simulink model "filter0"  (R2020b)
settings: Solver=FixedStepAuto  StartTime=0.0  StopTime=10.0  FixedStep=0.5  RelTol=1e-3
settings Model: Creator=Puru Gawande  LastModifiedBy=Puru Gawande
settings DataIOCC: SaveOutput=off  SaveTime=off

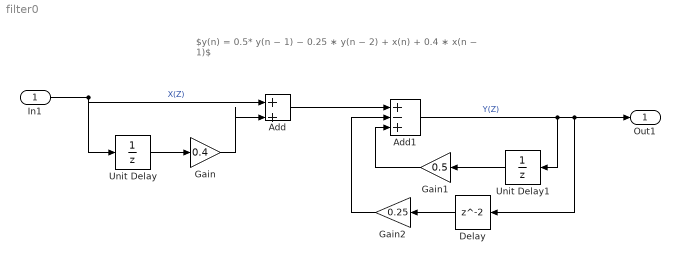
== system filter0 ==
  note: $y(n) = 0.5* y(n − 1) − 0.25 ∗ y(n − 2) + x(n) + 0.4 ∗ x(n − 1)$
  In1 : Inport  OutDataTypeStr=double  PortDimensions=[1 1]  SampleTime=[0.5,0]
  Add : Sum  Inputs=++|
  Add1 : Sum  Inputs=+-+
  Delay : Delay
  Gain : Gain  Gain=0.4
  Gain1 : Gain  Gain=0.5
  Gain2 : Gain  Gain=0.25
  Unit Delay : UnitDelay  SampleTime=-1  HasFrameUpgradeWarning=on
  Unit Delay1 : UnitDelay  SampleTime=-1  HasFrameUpgradeWarning=on
  Out1 : Outport  OutDataTypeStr=double  PortDimensions=1  SampleTime=[0.5,0]
  wires:
  Gain2/1 -> Add1/2
  In1/1 -> Add/1, Unit Delay/1  "X(Z)"
  Delay/1 -> Gain2/1
  Gain1/1 -> Add1/3
  Unit Delay/1 -> Gain/1
  Unit Delay1/1 -> Gain1/1
  Gain/1 -> Add/2
  Add/1 -> Add1/1
  Add1/1 -> Delay/1, Out1/1, Unit Delay1/1  "Y(Z)"
